simulink model "SmartHome"  (R2017a)
settings: Solver=VariableStepAuto  StartTime=0.0  StopTime=10.0  RelTol=1e-3
settings Model: Creator=Omid  LastModifiedBy=Omid

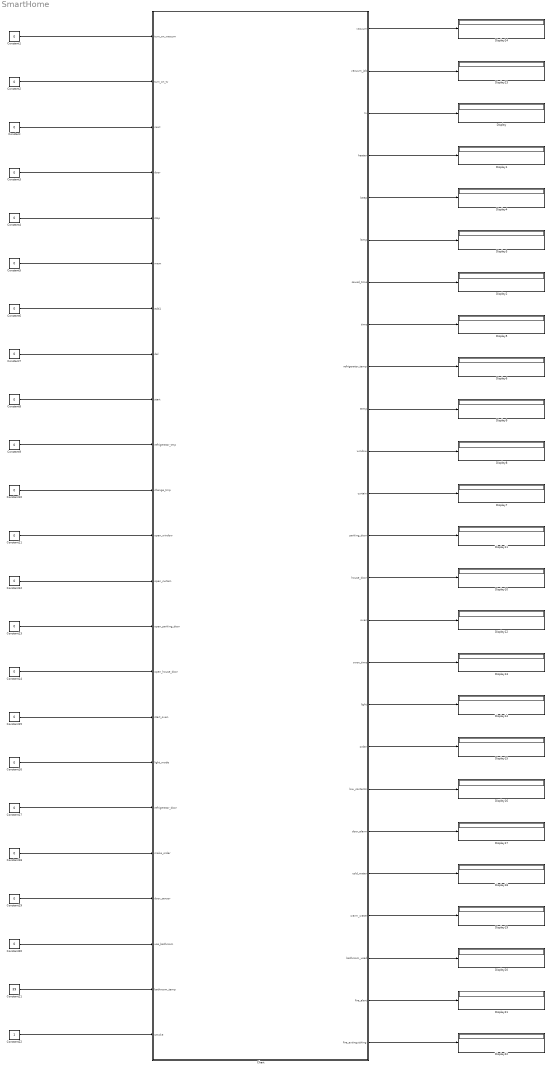
== system SmartHome ==
  Chart : Stateflow chart  TreatAsAtomicUnit=on
  Constant{,1..20} (21 alike) : Constant  Value=0
  Constant21 : Constant  Value=39
  Constant22 : Constant
  Display{,1..24} (25 alike) : Display
  wires:
  Constant1/1 -> Chart/1(turn_on_vaccum)
  Constant2/1 -> Chart/2(turn_on_tv)
  Constant8/1 -> Chart/9(start)
  Constant6/1 -> Chart/7(edit1)
  Constant7/1 -> Chart/8(del)
  Constant4/1 -> Chart/5(stop)
  Constant3/1 -> Chart/4(door)
  Constant5/1 -> Chart/6(mem)
  Constant/1 -> Chart/3(next)
  Chart/7(saved_time) -> Display2/1
  Chart/5(beep) -> Display4/1
  Chart/4(heater) -> Display1/1
  Chart/3(tv) -> Display/1
  Chart/8(time) -> Display5/1
  Chart/9(refrigerator_temp) -> Display6/1
  Constant9/1 -> Chart/10(refrigerator_tmp)
  Constant10/1 -> Chart/11(change_tmp)
  Constant11/1 -> Chart/12(open_window)
  Chart/10(temp) -> Display9/1
  Chart/11(window) -> Display8/1
  Chart/12(curtain) -> Display7/1
  Constant12/1 -> Chart/13(open_curtain)
  Constant13/1 -> Chart/14(open_parking_door)
  Constant14/1 -> Chart/15(open_house_door)
  Chart/6(lamp) -> Display3/1
  Chart/13(parking_door) -> Display11/1
  Chart/14(house_door) -> Display10/1
  Constant15/1 -> Chart/16(start_oven)
  Chart/15(oven) -> Display12/1
  Chart/16(oven_time) -> Display13/1
  Constant16/1 -> Chart/17(light_mode)
  Constant17/1 -> Chart/18(refrigerator_door)
  Constant18/1 -> Chart/19(make_order)
  Constant19/1 -> Chart/20(door_sensor)
  Chart/17(light) -> Display14/1
  Chart/18(order) -> Display15/1
  Chart/19(low_contents) -> Display16/1
  Chart/20(door_alarm) -> Display17/1
  Constant20/1 -> Chart/21(use_bathroom)
  Constant21/1 -> Chart/22(bathroom_temp)
  Chart/21(cold_water) -> Display18/1
  Chart/22(warm_water) -> Display19/1
  Chart/23(bathroom_used) -> Display20/1
  Constant22/1 -> Chart/23(smoke)
  Chart/24(fire_alart) -> Display21/1
  Chart/25(fire_extinguishing) -> Display22/1
  Chart/1(vacuum) -> Display24/1
  Chart/2(vacuum_job) -> Display23/1

== stateflow chart SmartHome/Chart ==
  state Controller
    state microwave_controller [parallel]
      settings: executionOrder=4
      state EditSec
        entry:
        sec = times(i) - floor(times(i)/60)
        saved_time = times(i);
      state AddMin
        entry:
        min=min+1;
      state SelectFromMem
        entry:
        saved_time = times(i);
        time = saved_time;
      state NextTime
        entry:
        i = i + 1;
      state AddMin2
        entry:
        min=min+1;
        sec = 0;
      state AddSec
        entry:
        sec=sec+1;
      state Open
        entry:
        heater = 0;
        lamp = 1;
        beep = 0;
      state EditMin
        entry:
        min = floor(times(i)/60)
        saved_time = times(i);
      state SaveTime
        entry:
        times(i)=sec+min*60;
        saved_time = times(i);
      state NextTime2
        entry:
        i = 0;
      state SelectMem
        entry:
        saved_time = times(i);
      state Pause
        entry:
        heater = 0;
        lamp = 0;
        beep = 0;
      state Init
        entry:
        time = 0;
        heater = 0;
        lamp = 0;
        beep = 0;
        times =  [0 0 0 0 0]
        i = 1;
      state Warm
        entry:
        time=time-1;
        heater = 1;
        lamp = 1;
        beep = 0;
      state Begin
        entry:
        time = 0;
        heater = 0;
        lamp = 0;
        beep = 0;
      state Start1
        entry:
        time = time + 5;
        heater = 1;
        lamp = 1;
        beep = 0;
      state Delete
        entry:
        times(i) = 0;
        saved_time = times(i);
      state End
        entry:
        time=0;
        heater = 0;
        lamp = 0;
        beep = 1;
        beep_counter = 3;
      state End1
        entry:
        time=0;
        heater = 0;
        lamp = 0;
        beep = 1;
        beep_counter = beep_counter - 1;
      EditSec -> AddSec : [next==1]
      NextTime -> SelectFromMem [order 1] : [start==1]
      AddMin -> AddMin [order 1] : [next==1]
      End -> Open [order 3] : [door==1]
      NextTime -> NextTime [order 5] : [next==1]
      AddMin -> EditSec [order 2] : [edit1==1]
      SelectMem -> SelectFromMem [order 2] : [start==1]
      EditMin -> EditSec [order 2] : [edit1==1]
      AddMin2 -> AddSec [order 1] : [next==1]
      SelectFromMem -> Warm
      EditMin -> AddMin [order 1] : [next==1]
      AddSec -> AddSec [order 1] : [next==1]
      AddSec -> AddMin2 [order 3] : [sec==60]
      NextTime -> EditMin [order 2] : [edit1==1]
      Pause -> Open [order 3] : [door==1]
      AddSec -> SaveTime [order 2] : [edit1==1]
      NextTime -> Delete [order 4] : [del == 1]
      AddMin2 -> SaveTime [order 2] : [edit1==1]
      Warm -> Open [order 4] : [door==1]
      End1 -> Open [order 2] : [door==1]
      Open -> Warm : [door==0 && start==1]
      NextTime -> NextTime2 [order 3] : [i==6]
      NextTime2 -> NextTime
      SelectMem -> NextTime [order 3] : [next==1]
      Start1 -> Open [order 3] : [door==1]
      Begin -> Open [order 3] : [door==1]
      SaveTime -> SelectMem
      (default) -> Init
      Warm -> Warm [order 5] : [time>0 && start==0 && stop==0 && door==0]
      Pause -> Warm [order 1] : [start==1]
      Begin -> SelectMem [order 4] : [mem==1]
      SelectMem -> Delete [order 4] : [del == 1]
      Delete -> SelectMem
      SelectMem -> Begin [order 1] : [mem==1]
      Warm -> Pause [order 3] : [stop==1]
      Pause -> Begin [order 2] : [stop==1]
      Start1 -> Pause [order 4] : [stop==1]
      Init -> Begin
      Warm -> End [order 2] : [time==0]
      Start1 -> Warm [order 2] : [time>0 && start==0 && stop==0 && door==0]
      Start1 -> Start1 [order 1] : [start==1]
      Warm -> Start1 [order 1] : [start==1]
      Begin -> Begin [order 1] : [stop==1]
      Begin -> Start1 [order 2] : [start==1]
      End1 -> Begin [order 1] : [start==1 | stop==1 | beep_counter==0]
      End -> Begin [order 1] : [start==1 | stop==1]
      End1 -> End1 [order 3] : [start==0 && stop==0 && door==0]
      End -> End1 [order 2] : [start==0 && stop==0 && door==0]
    state vacuum_controller [parallel]
      settings: executionOrder=2
      state vacuum_off
        entry: vacuum=0;
      state vacuum_on
        entry: vacuum=1;
        vacuum_time=vacuum_time-1;
        vacuum_job=1;
      state vacuum_finish
        entry: vacuum_time=5;
        vacuum=0;
        vacuum_job=0;
      (default) -> vacuum_off
      vacuum_off -> vacuum_on : [turn_on_vaccum==1]
      vacuum_finish -> vacuum_off : [vacuum==0]
      vacuum_on -> vacuum_off [order 2] : [turn_on_vaccum==0]
      vacuum_on -> vacuum_finish [order 1] : [vacuum_time==0]
      vacuum_on -> vacuum_on [order 3] : [vacuum_time>0]
    state tv_controller [parallel]
      settings: executionOrder=1
      state tv_off
        entry: tv=0;
      state tv_on
        entry: tv=1;
        if smoke==1
        tv=0
        end
      tv_off -> tv_on : [turn_on_tv==1]
      (default) -> tv_off
      tv_on -> tv_on [order 2] : [turn_on_tv==1]
      tv_on -> tv_off [order 1] : [turn_on_tv==0 | house_door==1]
    state window_controller [parallel]
      settings: executionOrder=6
      state window_close
        entry: window=0;
        if smoke==1
        window=1
        end
      state window_open
        entry: window=1;
      (default) -> window_close
      window_close -> window_open [order 1] : [open_window==1]
      window_close -> window_close [order 2] : [open_window==0]
      window_open -> window_close : [open_window==0]
    state heater_controller [parallel]
      settings: executionOrder=5
      state heater_config
        entry:
      state tmp_up
        entry:
        temp=temp+1;
        if temp == 36
        temp=35;
        end
      state tmp_down
        entry:
        temp=temp-1;
        if temp == 19
        temp=20;
        end
      tmp_up -> tmp_up [order 2] : [change_tmp==1]
      (default) -> heater_config
      heater_config -> tmp_up [order 1] : [change_tmp==1]
      tmp_down -> tmp_up [order 1] : [change_tmp==1]
      tmp_up -> tmp_down [order 1] : [change_tmp==2]
      heater_config -> tmp_down [order 2] : [change_tmp==2]
      tmp_down -> tmp_down [order 2] : [change_tmp==2]
    state door_controller [parallel]
      settings: executionOrder=8
      state door_close
        entry: house_door=0;
      state door_open
        entry: house_door=1;
      (default) -> door_close
      door_close -> door_open : [open_house_door==1]
      door_open -> door_close : [open_house_door==0]
    state bathroom_controller [parallel]
      settings: executionOrder=13
      state bathroom_close
        entry:
        cold_water=0;
        warm_water=0;
        bathroom_used=0;
      state bathroom_open
        entry:
        if bathroom_temp>=40
        cold_water=1;
        warm_water=0;
        end
        if bathroom_temp<=20
        cold_water=0;
        warm_water=1;
        end
        if bathroom_temp<40 && bathroom_temp>20
        cold_water=0;
        warm_water=0;
        end
        bathroom_used=1;
      bathroom_open -> bathroom_open [order 2] : [use_bathroom==1]
      (default) -> bathroom_close
      bathroom_close -> bathroom_open : [use_bathroom==1]
      bathroom_open -> bathroom_close [order 1] : [use_bathroom==0]
    state parking_door_controller [parallel]
      settings: executionOrder=9
      state parking_door_close
        entry: parking_door=0;
      state parking_door_open
        entry: parking_door=1;
      (default) -> parking_door_close
      parking_door_close -> parking_door_open : [open_parking_door==1]
      parking_door_open -> parking_door_close : [open_parking_door==0]
    state curtain_controller [parallel]
      settings: executionOrder=7
      state curtain_close
        entry: curtain=0;
      state curtain_open
        entry: curtain=1;
      (default) -> curtain_close
      curtain_close -> curtain_open : [open_curtain==1]
      curtain_open -> curtain_close : [open_curtain==0|tv==1|open_house_door==1]
    state oven_controller [parallel]
      settings: executionOrder=10
      state oven_start
        entry: oven=0;
        oven_time=0;
      state oven_stop
        entry: oven=1;
        if smoke==1
        oven=0
        else
        oven_time=oven_time+1
        end
      (default) -> oven_start
      oven_start -> oven_stop : [start_oven==1]
      oven_stop -> oven_start [order 1] : [start_oven==0]
      oven_stop -> oven_stop [order 2] : [start_oven==1]
    state door_alarm_controller [parallel]
      settings: executionOrder=12
      state door_not_alarm
        entry: door_alarm=0;
      state door_alarm1
        entry: door_alarm=1;
      (default) -> door_not_alarm
      door_not_alarm -> door_alarm1 : [door_sensor==1]
      door_alarm1 -> door_not_alarm : [door_sensor==0]
    state light_controller [parallel]
      settings: executionOrder=11
      state light0
        entry: light=0;
      state light1
        entry: light=1;
      state light2
        entry: light=2;
      (default) -> light0
      light0 -> light1 [order 1] : [light_mode==1|tv==1]
      light1 -> light0 [order 2] : [light_mode==0]
      light0 -> light2 [order 2] : [light_mode==2]
      light2 -> light0 [order 1] : [light_mode==0]
      light2 -> light1 [order 2] : [light_mode==1|tv==1]
      light1 -> light2 [order 1] : [light_mode==2]
    state refrigerator_controller [parallel]
      settings: executionOrder=3
      state refrigerator_door_opened
        entry:
        contents=contents-1;
        if contents <= 5 && make_order==1
        low_contents =1;
        order=1;
        elseif contents <= 5 && make_order~=1
        low_contents =1;
        order=0;
        else
        low_contents =0;
        order=0;
        end
      state refrigerator_up
        entry:
        refrigerator_temp=refrigerator_temp+1;
        if refrigerator_temp == 21
        refrigerator_temp=20;
        end
        if contents <= 5 && make_order==1
        low_contents =1;
        order=1;
        elseif contents <= 5 && make_order~=1
        low_contents =1;
        order=0;
        else
        low_contents =0;
        order=0;
        end
      state refrigerator_init
        entry:
        if contents <= 5 && make_order==1
        low_contents =1;
        order=1;
        elseif contents <= 5 && make_order~=1
        low_contents =1;
        order=0;
        else
        low_contents =0;
        order=0;
        end
      state refrigerator_down
        entry:
        refrigerator_temp=refrigerator_temp-1;
        if refrigerator_temp == -11
        refrigerator_temp=-10;
        end
        if contents <= 5 && make_order==1
        low_contents =1;
        order=1;
        elseif contents <= 5 && make_order~=1
        low_contents =1;
        order=0;
        else
        low_contents =0;
        order=0;
        end
      refrigerator_door_opened -> refrigerator_door_opened [order 2] : [refrigerator_door==1]
      refrigerator_up -> refrigerator_up [order 2] : [refrigerator_tmp==1]
      refrigerator_up -> refrigerator_door_opened [order 3] : [refrigerator_door==1]
      refrigerator_init -> refrigerator_init [order 4] : [refrigerator_tmp==0]
      refrigerator_init -> refrigerator_door_opened [order 3] : [refrigerator_door==1]
      (default) -> refrigerator_init
      refrigerator_init -> refrigerator_up [order 1] : [refrigerator_tmp==1]
      refrigerator_door_opened -> refrigerator_init [order 1] : [refrigerator_door==0]
      refrigerator_down -> refrigerator_door_opened [order 3] : [refrigerator_door==1]
      refrigerator_up -> refrigerator_init [order 4] : [refrigerator_tmp==0]
      refrigerator_down -> refrigerator_up [order 1] : [refrigerator_tmp==1]
      refrigerator_up -> refrigerator_down [order 1] : [refrigerator_tmp==2]
      refrigerator_down -> refrigerator_init [order 4] : [refrigerator_tmp==0]
      refrigerator_init -> refrigerator_down [order 2] : [refrigerator_tmp==2]
      refrigerator_down -> refrigerator_down [order 2] : [refrigerator_tmp==2]
    state fire_controller [parallel]
      settings: executionOrder=14
      state fire_detect
        entry: fire_alart=0;
        fire_extinguishing=0;
      state fire_not_detect
        entry: fire_alart=1;
        fire_extinguishing=1;
      (default) -> fire_detect
      fire_detect -> fire_not_detect : [smoke==1]
      fire_not_detect -> fire_detect : [smoke==0]
  state Start
    entry:
    vacuum=0;
    vacuum_time=5;
    vacuum_job=0;
    tv=0;
    refrigerator_temp=5;
    temp=30;
    window=0;
    curtain=0;
    house_door=0;
    parking_door=0;
    oven=0;
    oven_time=0;
    light=0;
    contents=10;
    door_alarm=0;
    cold_water=0;
    warm_water=0;
    bathroom_used=0;
  (default) -> Start
  Start -> Controller
  data: turn_on_vaccum input; vacuum output; vacuum_time local; vacuum_job output; turn_on_tv input; tv output; next input; door input; stop input; mem input; edit1 input; del input; start input; heater output; beep output; lamp output; beep_counter local; i local; min local; sec local; times local; saved_time output; time output; refrigerator_temp output; refrigerator_tmp input; change_tmp input; temp output; open_window input; window output; open_curtain input; curtain output; open_parking_door input; parking_door output; open_house_door input; house_door output; start_oven input; oven output; oven_time output; light_mode input; light output; refrigerator_door input; make_order input; order output; low_contents output; contents local; door_sensor input; door_alarm output; use_bathroom input; bathroom_temp input; cold_water output; warm_water output; bathroom_used output; smoke input; fire_alart output; fire_extinguishing output
